simulink model "StarshotAC_DC_kd12"  (R2017a)
settings: Solver=FixedStepAuto  StartTime=0  StopTime=50000  FixedStep=0.01  MaxStep=4.0  MinStep=.001  RelTol=1e-6
values from neighbouring files (symbols this model uses):
  B0 = 3.12e-5    (= 3.12e-05)    [starshot_DC_KD_setup.m]    (also in starshot_DC_setup.m; starshotmath.m; temp.m)
  G = 6.67e-11    [starshot_DC_KD_setup.m]    (also in starshot_DC_setup.m; temp.m)
  M_Earth = 5.972e24    (= 5.972e+24)    [starshot_DC_KD_setup.m]    (also in starshot_DC_setup.m; temp.m)
  q0 = [qmatlab(2:4),qmatlab(1)]'    [starshot_DC_KD_setup.m]    (also in starshot_DC_setup.m; temp.m)
  R_Earth = 6.378e6    (= 6378000)    [starshot_DC_KD_setup.m]    (also in starshot_DC_setup.m; temp.m)
undefined symbols (not defined in the file or in its folder): starshot
libraries: dspmathops x1, sharedtransform x1, simulink x1
settings Model: Creator=armen  LastModifiedBy=Davide

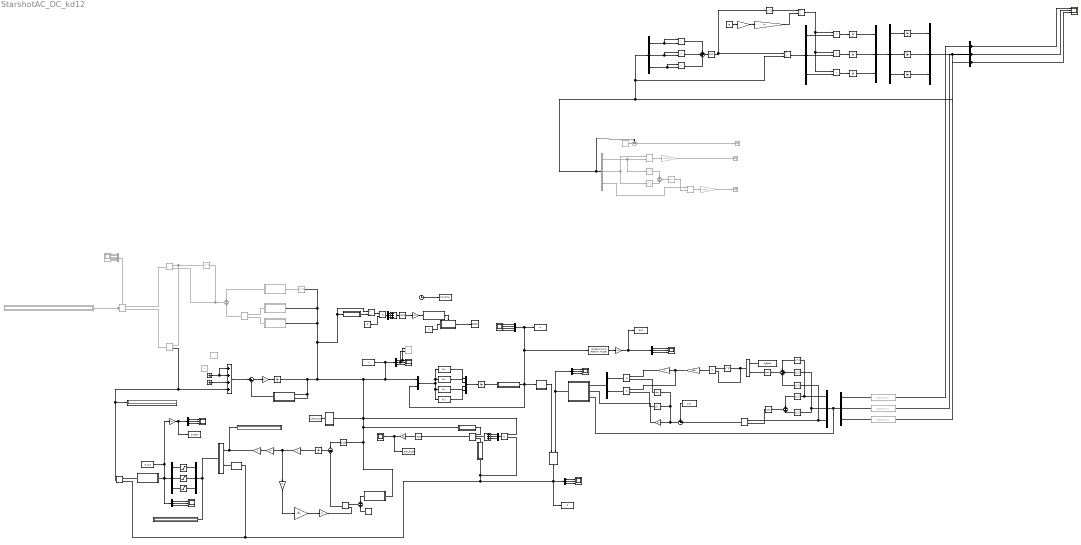
== system StarshotAC_DC_kd12 ==
  note: Dynamics
  note: Kynematics
  note: Earth's magnetic dipole
  note: Magnetic dipole/torque
  (w_b)x(L_b) : Subsystem
  Add : Sum  Inputs=3
  Add1 : Sum  Inputs=+++
  Angular velocity : Scope  NumInputPorts=3
  Clock : Clock
  Constant : Constant  Value=-G
  Constant1 : Constant  Value=R_Earth
  Constant2 : Constant  Commented=on  Value=[0;0;0]
  Constant3 : Constant  Value=starshot.IC.massproperties.PI(:,3)'
  Constant4 : Constant
  Constant5 : Constant  Commented=on  Value=starshot.IC.x
  Constant6 : Constant  Commented=on  Value=starshot.IC.y
  Constant7 : Constant  Commented=on  Value=starshot.IC.z
  Constant8 : Constant  Value=pi/2
  Cross : Subsystem
  Current : Scope  NumInputPorts=3
  Demux{,1..5,7..10,12,14,16,18} (14 alike) : Demux  Outputs=3
  Demux11 : Demux  Commented=on  Outputs=6
  Demux13 : Demux
  Demux6 : Demux  Commented=on  Outputs=3
  Derivative : Derivative
  Derivative1 : Derivative  Commented=on
  Dipole->ECI : Subsystem
  Display : Display  Commented=on
  Display1 : Display
  Display4 : Display
  Display6 : Display
  Divide : Product  Inputs=/*
  Divide1 : Product  Inputs=/*
  Divide2 : Product  Inputs=*/
  Divide3 : Product  Inputs=**
  Divide4 : Product  Inputs=**
  Divide5 : Product  Commented=on  Inputs=/*  Multiplication=Matrix(*)
  Divide6 : Product  Inputs=/*/
  Dot Product{,1..5} (6 alike) : DotProduct  InputSameDT=on  OutDataTypeStr=Inherit: Inherit via internal rule
  Earth's magnetic field (ECI) : Scope  NumInputPorts=3
  Earth's magnetic field (body) : Scope  NumInputPorts=3
  Euler angles : Scope  NumInputPorts=3
  Gain : Gain  Commented=on  Gain=180/pi
  Gain 1 : Gain  SaturateOnIntegerOverflow=on  OutDataTypeStr=Inherit: Same as input  ParamDataTypeStr=Inherit: Same as input
  Gain 2 : Gain  Gain=-1  SaturateOnIntegerOverflow=on  OutDataTypeStr=Inherit: Same as input  ParamDataTypeStr=Inherit: Same as input
  Gain 8 : Gain  Gain=starshot.cmd.c  SaturateOnIntegerOverflow=on  OutDataTypeStr=Inherit: Same as input  ParamDataTypeStr=Inherit: Same as input
  Gain 9 : Gain  Gain=-1  SaturateOnIntegerOverflow=on  OutDataTypeStr=Inherit: Same as input  ParamDataTypeStr=Inherit: Same as input
  Gain1 : Gain  Gain=M_Earth
  Gain18 : Gain  Gain=180/pi
  Gain2 : Gain  Gain=starshot.IC.massproperties.m
  Gain3 : Gain  Commented=on  Gain=180/pi
  Gain4 : Gain  Gain=-B0
  Gain5 : Gain  Gain=2
  Gain6 : Gain  Gain=-1
  Gain7 : Gain  Gain=1/0.0005
  Gain8 : Gain  Gain=180/pi
  Gain9 : Gain  Gain=180/pi
  Id inverse : Gain  Gain=starshot.cmd.invId  Multiplication=Matrix(K*u)  SaturateOnIntegerOverflow=on  OutDataTypeStr=Inherit: Same as input  ParamDataTypeStr=Inherit: Same as input
  Identity matrix : Constant  Value=[1 0 0;0 1 0;0 0 1]
  If : If  IfExpression=u1 < 0.2| u1>179.8  ShowElse=off
  If Action Subsystem : Subsystem  TreatAsAtomicUnit=on
  Integrator : Integrator  InitialCondition=starshot.IC.x
  Integrator1 : Integrator  InitialCondition=starshot.IC.y
  Integrator2 : Integrator  InitialCondition=starshot.IC.z
  Integrator3 : Integrator  InitialCondition=starshot.IC.xdot
  Integrator4 : Integrator  InitialCondition=starshot.IC.ydot
  Integrator5 : Integrator  InitialCondition=starshot.IC.zdot
  Integrator6 : Integrator  InitialCondition=starshot.IC.w
  Integrator7 : Integrator  InitialCondition=q0
  Integrator8 : Integrator  InitialCondition=starshot.cmd.wdb0
  Inv(I) : Gain  Gain=starshot.IC.massproperties.Iinv  Multiplication=Matrix(K*u)
  Kane damping : Gain  Gain=starshot.cmd.c  SaturateOnIntegerOverflow=on  OutDataTypeStr=Inherit: Same as input  ParamDataTypeStr=Inherit: Same as input
  L : Subsystem  Commented=on
  L1 : Subsystem  Commented=on
  Math Function{,3..8} (7 alike) : Math  Operator=square  SaturateOnIntegerOverflow=on
  Math Function1 : Math  Commented=on  Operator=square  SaturateOnIntegerOverflow=on
  Math Function2 : Math  Commented=on  Operator=square  SaturateOnIntegerOverflow=on
  Math Function9 : Math  Commented=on  Operator=transpose  SaturateOnIntegerOverflow=on
  Matrix Multiply : Product  Multiplication=Matrix(*)
  Mux{,1,6,9} (4 alike) : Mux  Inputs=3
  Mux10 : Mux
  Mux3 : Mux  Inputs=2
  Mux4 : Mux  Inputs=2
  Norm1 : Subsystem
  Norm4 : Subsystem
  Norm5 : Subsystem
  Normalization : dspmathops/Normalization  NormType=Squared 2-norm  Bias=1e-10  NormOver=Each column  Dimension=1  outputDataTypeStr=Inherit: Same as product output  outputLastDataTypeStr=Inherit: Same as product output  outputMin=[]  outputMax=[]  accumDataTypeStr=Inherit: Same as product output  accumLastDataTypeStr=Inherit: Same as product output  roundingMode=Floor  overflowMode=off
      settings: SourceProductName=DSP System Toolbox
  Normalized quat : Subsystem
  Product : Product
  Product1 : Product  Multiplication=Matrix(*)
  Product2 : Product  Multiplication=Matrix(*)
  Product3 : Product  Commented=on  Multiplication=Matrix(*)
  Product4 : Product  Commented=on  Multiplication=Matrix(*)
  Product5 : Product  Commented=on  Multiplication=Matrix(*)
  Product6 : Product
  Product7 : Product  Inputs=*/
  Product8 : Product
  Quaternion : Scope  NumInputPorts=4
  Quaternions to Rotation Angles : sharedtransform/Quaternions to Rotation Angles  rotationOrder=ZYX
  R_earth : Constant  Commented=on  Value=6.371e6
  Saturation : Saturate  UpperLimit=starshot.magnetorq.m_max_x  LowerLimit=-starshot.magnetorq.m_max_x
  Saturation1 : Saturate  UpperLimit=starshot.magnetorq.m_max_y  LowerLimit=-starshot.magnetorq.m_max_y
  Saturation2 : Saturate  UpperLimit=starshot.magnetorq.m_max_z  LowerLimit=-starshot.magnetorq.m_max_z
  Scope : Scope  NumInputPorts=3
  Scope1 : Scope  Commented=on  NumInputPorts=6
  Scope2 : Scope
  Skew matrix S(m) : Subsystem
  Skew matrix S(m)1 : Subsystem
  Skew matrix S(w) : Subsystem  Commented=on
  Sqrt : Sqrt  SaturateOnIntegerOverflow=on
  Sqrt1 : Sqrt  Commented=on  SaturateOnIntegerOverflow=on
  Sqrt2 : Sqrt  SaturateOnIntegerOverflow=on
  Sqrt3 : Sqrt  SaturateOnIntegerOverflow=on
  Stop Simulation : Stop
  Subsystem : Subsystem
  Sum : Sum  Inputs=+++
  Sum1 : Sum  Commented=on  Inputs=+-|
  Sum10 : Sum  Inputs=+|+  SaturateOnIntegerOverflow=on  InputSameDT=on  OutDataTypeStr=Inherit: Same as first input
  Sum12 : Sum  Inputs=|+-
  Sum2 : Sum  Commented=on
  Sum3 : Sum
  Sum4 : Sum  Inputs=+++
  Sum5 : Sum  Inputs=+-|
  Sum6 : Sum  Inputs=++++
  Sum7 : Sum  Commented=on  Inputs=+|+
  Sum8 : Sum  Inputs=--
  T_aero : Constant  Commented=on  Value=-starshot.aerodrag.Ta
  T_gravity : Ground
  T_solar : Ground
  Terminator : Terminator  Commented=on
  Terminator1 : Terminator  Commented=on
  Terminator2 : Terminator  Commented=on
  To Workspace : ToWorkspace  VariableName=real_angle  SaveFormat=Timeseries  SampleTime=-1
  To Workspace1 : ToWorkspace  VariableName=w  SaveFormat=Timeseries  SampleTime=-1
  To Workspace2 : ToWorkspace  VariableName=Eul1  SaveFormat=Timeseries  SampleTime=-1
  To Workspace3 : ToWorkspace  VariableName=w_error_out  SaveFormat=Timeseries  SampleTime=-1
  To Workspace4 : ToWorkspace  VariableName=b  SaveFormat=Timeseries  SampleTime=-1
  To Workspace5 : ToWorkspace  VariableName=m_out  SaveFormat=Timeseries  SampleTime=-1
  To Workspace6 : ToWorkspace  VariableName=q  SaveFormat=Timeseries  SampleTime=-1
  To Workspace7 : ToWorkspace  VariableName=current  SaveFormat=Timeseries  SampleTime=-1
  To Workspace8 : ToWorkspace  VariableName=sim_time  SaveFormat=Timeseries  SampleTime=-1
  Trigonometric Function : Trigonometry  Commented=on  Operator=atan2
  Trigonometric Function1 : Trigonometry  Commented=on  Operator=atan2
  Trigonometric Function2 : Trigonometry  Operator=cos
  Trigonometric Function3 : Trigonometry  Operator=atan2
  Trigonometric Function4 : Trigonometry
  Trigonometric Function5 : Trigonometry  Operator=acos
  Trigonometric Function6 : Trigonometry  Operator=acos
  XY Graph : simulink/Sinks/XY Graph  Commented=on  xmin=-2  xmax=2  ymin=-2  ymax=2  st=-1
  magnetic dipole : Scope  NumInputPorts=3
  qd(0) : Fcn  Expr=(u(7)*u(1)-u(6)*u(2)+u(5)*u(3))/2
  qd(1) : Fcn  Expr=(u(6)*u(1)+u(7)*u(2)-u(4)*u(3))/2
  qd(2) : Fcn  Expr=(-u(5)*u(1)+u(4)*u(2)+u(7)*u(3))/2
  qd(3) : Fcn  Expr=(-u(4)*u(1)-u(5)*u(2)-u(6)*u(3))/2
  quat to DCM : Subsystem  mask(Direction Cosine Matrix){}
      mask help: Determines the 3x3 Direction Cosine Matrix (DCM) from a 4x1 quaternion orientation vector. The outputted DCM transforms vectors from inertial axes to body axes. This version corrects the fucked-up MATLAB one.
      mask Help:
      | <p>This block determines the 3x3 Direction Cosine Matrix (DCM) from a 4x1 quaternion orientation vector. The outputted DCM transforms vectors from inertial axes to body axes.  This version corrects the fucked-up MATLAB one</p>
      | 
      | <p>The block input and output contain more than one signal as described below.</p>
      | 
      | <p><H4>Block Vector Input - Quaternion</H4>
      | <ul>
      | <li>q0</li>
      | <li>q1</li>
      | <li>q2</li>
      | <li>q3</li>
      | </ul>
      | </p>
      | 
      | <p><H4>Block Matrix Output - Direction Cosine Matrix  </H4>
      |     <ul>
      |    </ul>
      |    </p>
      mask Display: disp('q to Q')
  wires:
  Integrator/1 -> Mux/1
  Integrator2/1 -> Mux/3
  Integrator1/1 -> Mux/2
  Demux/3 -> Integrator2/1
  Demux/2 -> Integrator1/1
  Demux/1 -> Integrator/1
  Mux1/1 -> Demux/1
  Integrator5/1 -> Mux1/3
  Integrator4/1 -> Mux1/2
  Integrator3/1 -> Mux1/1
  Demux1/1 -> Dot Product/1, Dot Product/2
  Demux1/2 -> Dot Product1/1, Dot Product1/2
  Demux1/3 -> Dot Product2/1, Dot Product2/2
  Dot Product1/1 -> Sum/2
  Dot Product2/1 -> Sum/3
  Dot Product/1 -> Sum/1
  Sum/1 -> Sqrt/1
  Constant/1 -> Gain1/1
  Sqrt/1 -> Math Function/1, Divide1/1
  Gain1/1 -> Gain2/1
  Gain2/1 -> Divide/2
  Math Function/1 -> Divide/1
  Divide/1 -> Dot Product3/1, Dot Product4/1, Dot Product5/1
  Demux2/3 -> Dot Product3/2
  Demux2/2 -> Dot Product4/2
  Demux2/1 -> Dot Product5/2
  Dot Product5/1 -> Integrator3/1
  Dot Product4/1 -> Integrator4/1
  Dot Product3/1 -> Integrator5/1
  Divide1/1 -> Demux2/1
  Sum1/1 -> Terminator/1
  R_earth/1 -> Sum1/2
  Demux6/1 -> Math Function2/1, Trigonometric Function/2
  Demux6/2 -> Trigonometric Function/1, Math Function1/1
  Demux6/3 -> Trigonometric Function1/1
  Math Function2/1 -> Sum2/1
  Math Function1/1 -> Sum2/2
  Sum2/1 -> Sqrt1/1
  Sqrt1/1 -> Trigonometric Function1/2
  Trigonometric Function/1 -> Gain/1
  Trigonometric Function1/1 -> Gain3/1
  Gain/1 -> Terminator1/1
  Gain3/1 -> Terminator2/1
  Sqrt2/1 -> Trigonometric Function3/2
  Sum3/1 -> Sqrt2/1
  Math Function3/1 -> Sum3/2
  Math Function4/1 -> Sum3/1
  Demux7/3 -> Math Function7/1, Trigonometric Function3/1
  Demux7/2 -> Math Function3/1, Math Function6/1
  Demux7/1 -> Math Function5/1, Math Function4/1
  Mux/1 -> Sum1/1, Demux6/1, Divide1/2, Demux1/1, Demux3/1
  Math Function6/1 -> Sum4/2
  Math Function5/1 -> Sum4/1
  Math Function7/1 -> Sum4/3
  Sum4/1 -> Sqrt3/1
  Sqrt3/1 -> Divide2/2
  Constant1/1 -> Divide2/1
  Divide2/1 -> Product/2, Math Function8/1
  Math Function8/1 -> Product/1
  Product/1 -> Gain4/1
  Gain4/1 -> Divide4/1, Gain5/1
  Gain5/1 -> Divide3/1
  Trigonometric Function2/1 -> Divide3/2
  Trigonometric Function4/1 -> Divide4/2
  Divide3/1 -> Mux4/1
  Divide4/1 -> Mux4/2
  Mux4/1 -> Dipole->ECI/1(B_r,B_theta)
  Gain6/1 -> Dipole->ECI/2(-theta)
  Demux9/3 -> Earth's magnetic field (ECI)/3
  Demux9/1 -> Earth's magnetic field (ECI)/1
  Demux9/2 -> Earth's magnetic field (ECI)/2
  Mux6/1 -> Dipole->ECI/3(r), Demux7/1
  Demux3/3 -> Scope/3, Mux6/3
  Demux3/2 -> Scope/2, Mux6/2
  Demux3/1 -> Scope/1, Mux6/1
  Trigonometric Function3/1 -> Sum5/2
  Constant8/1 -> Sum5/1
  Sum5/1 -> Trigonometric Function2/1, Trigonometric Function4/1, Gain6/1
  Demux13/1 -> Quaternion/1
  Demux13/4 -> Quaternion/4
  Demux13/3 -> Quaternion/3
  Demux13/2 -> Quaternion/2
  Demux16/2 -> XY Graph/2, Angular velocity/2
  Demux16/1 -> XY Graph/1, Angular velocity/1
  Demux16/3 -> Angular velocity/3
  Dipole->ECI/1(B) -> Demux9/1, Matrix Multiply/2
  Demux8/1 -> Saturation/1
  Saturation2/1 -> Mux9/3
  Saturation/1 -> Mux9/1
  Demux8/2 -> Saturation1/1
  Saturation1/1 -> Mux9/2
  Demux10/3 -> magnetic dipole/3
  Demux10/2 -> magnetic dipole/2
  Demux10/1 -> magnetic dipole/1
  quat to DCM/1(DCM) -> Matrix Multiply/1
  Demux18/3 -> Euler angles/3
  Demux18/1 -> Euler angles/1
  Gain18/1 -> To Workspace2/1, Demux18/1  "Euler Angles plot"
  Quaternions to Rotation Angles/1 -> Gain18/1
  Demux18/2 -> Euler angles/2
  Inv(I)/1 -> Integrator6/1
  (w_b)x(L_b)/1((w_b)x(L_b)) -> Sum12/2
  Sum12/1 -> Inv(I)/1  "wdot"
  qd(2)/1 -> Mux10/3
  qd(1)/1 -> Mux10/2
  Normalized quat/1(q^) -> Mux3/2, quat to DCM/1(e0 e1 e2 e3), Quaternions to Rotation Angles/1, To Workspace6/1, Demux13/1  "q^"
  qd(3)/1 -> Mux10/4
  Integrator7/1 -> Normalized quat/1(q)
  Mux10/1 -> Integrator7/1
  qd(0)/1 -> Mux10/1
  Mux3/1 -> qd(3)/1, qd(2)/1, qd(1)/1, qd(0)/1
  Demux4/1 -> Earth's magnetic field (body)/1
  Demux4/2 -> Earth's magnetic field (body)/2
  Demux4/3 -> Earth's magnetic field (body)/3
  T_gravity/1 -> Sum6/1, Sum6/2
  Sum6/1 -> Sum12/1
  Mux9/1 -> Skew matrix S(m)/1(m), To Workspace5/1, Gain7/1, Demux10/1
  Gain7/1 -> To Workspace7/1, Demux5/1
  Demux5/1 -> Current/1
  Demux5/2 -> Current/2
  Demux5/3 -> Current/3
  Skew matrix S(m)/1(S(m)) -> Product2/1
  Demux8/3 -> Saturation2/1
  Cross/1(AxB) -> Display6/1, Demux8/1
  Product2/1 -> Product4/2, Sum6/4, Display4/1
  Gain 2/1 -> Kane damping/1, Gain 9/1
  Normalization/1 -> Cross/2(B)
  Kane damping/1 -> Gain 1/1
  Derivative/1 -> Sum8/1
  Sum8/1 -> Integrator8/1
  Gain 8/1 -> Product1/2
  Id inverse/1 -> Gain 8/1
  Skew matrix S(m)1/1(S(w)) -> Sum10/1
  Identity matrix/1 -> Sum10/2
  Gain 9/1 -> Id inverse/1
  Sum10/1 -> Product1/1
  Product1/1 -> Sum8/2
  Gain 1/1 -> Display1/1, Cross/1(A)
  Integrator8/1 -> Gain 2/1  "w_(d/b)"
  Divide5/1 -> Display/1, Demux11/1
  Sum7/1 -> Product3/2, Math Function9/1
  Math Function9/1 -> Product4/1, Product3/1
  Product3/1 -> Divide5/1
  Product4/1 -> Divide5/2
  Demux11/1 -> Scope1/1
  Demux11/2 -> Scope1/2
  Demux11/3 -> Scope1/3
  Demux11/4 -> Scope1/4
  Demux11/5 -> Scope1/5
  Demux11/6 -> Scope1/6
  L1/1(L(a)) -> Product5/2
  Skew matrix S(w)/1(S(w)) -> Product5/1
  L/1(L(a)) -> Sum7/1
  Product5/1 -> Sum7/2
  Derivative1/1 -> L/1(a)
  Demux12/3 -> Add/3
  Divide6/1 -> Trigonometric Function5/1
  Norm5/1(norm(v)) -> Divide6/3
  Add/1 -> Divide6/2
  Matrix Multiply/1 -> To Workspace4/1, Demux4/1, Product6/2, Norm5/1(v), Normalization/1, Product2/2
  Demux12/1 -> Add/1
  Demux12/2 -> Add/2
  Integrator6/1 -> Product7/1, Norm1/1(v), Derivative1/1, Skew matrix S(w)/1(w), L1/1(a), Subsystem/1(In1), Norm4/1(v), Skew matrix S(m)1/1(w), Derivative/1, Product6/1, Mux3/1, Demux16/1, To Workspace1/1, (w_b)x(L_b)/2(L_b), (w_b)x(L_b)/1(w_b)  "w"
  Product6/1 -> Demux12/1
  Trigonometric Function5/1 -> Gain8/1
  Norm4/1(norm(v)) -> Divide6/1
  Gain8/1 -> To Workspace/1, Scope2/1
  Subsystem/1(Out1) -> To Workspace3/1
  T_solar/1 -> Sum6/3
  Constant3/1 -> Product8/2
  Norm1/1(norm(v)) -> Product7/2
  Trigonometric Function6/1 -> Gain9/1
  Gain9/1 -> If/1
  Product7/1 -> Product8/1
  If/1 -> If Action Subsystem/Action
  Constant4/1 -> If Action Subsystem/1(In1)
  If Action Subsystem/1(Out1) -> Stop Simulation/1
  Add1/1 -> Trigonometric Function6/1
  Product8/1 -> Demux14/1
  Demux14/1 -> Add1/1
  Demux14/2 -> Add1/2
  Demux14/3 -> Add1/3
  Clock/1 -> To Workspace8/1

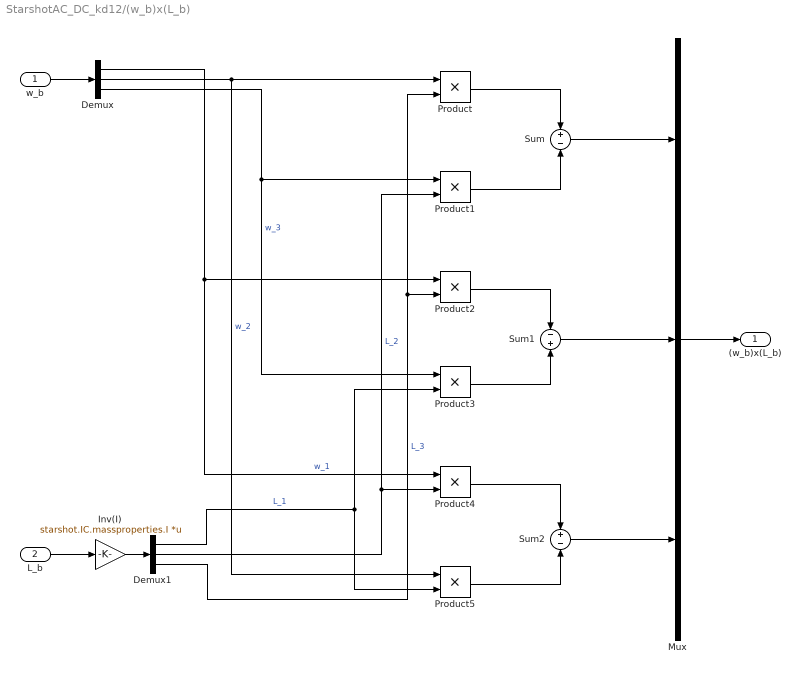
== system StarshotAC_DC_kd12/(w_b)x(L_b) ==
  w_b : Inport
  L_b : Inport  Port=2
  Demux : Demux  Outputs=3
  Demux1 : Demux  Outputs=3
  Inv(I) : Gain  Gain=starshot.IC.massproperties.I  Multiplication=Matrix(K*u)
  Mux : Mux  Inputs=3
  Product{,1..5} (6 alike) : Product
  Sum : Sum  Inputs=+|-
  Sum1 : Sum  Inputs=-|+
  Sum2 : Sum  Inputs=+|-
  (w_b)x(L_b) : Outport
  wires:
  w_b/1 -> Demux/1
  L_b/1 -> Inv(I)/1
  Demux/3 -> Product1/1, Product3/1  "w_3"
  Demux/2 -> Product5/1, Product/1  "w_2"
  Demux/1 -> Product2/1, Product4/1  "w_1"
  Mux/1 -> (w_b)x(L_b)/1
  Demux1/3 -> Product2/2, Product/2  "L_3"
  Demux1/2 -> Product1/2, Product4/2  "L_2"
  Product1/1 -> Sum/2
  Product/1 -> Sum/1
  Demux1/1 -> Product5/2, Product3/2  "L_1"
  Sum/1 -> Mux/1
  Sum2/1 -> Mux/3
  Sum1/1 -> Mux/2
  Product5/1 -> Sum2/2
  Product4/1 -> Sum2/1
  Product3/1 -> Sum1/2
  Product2/1 -> Sum1/1
  Inv(I)/1 -> Demux1/1

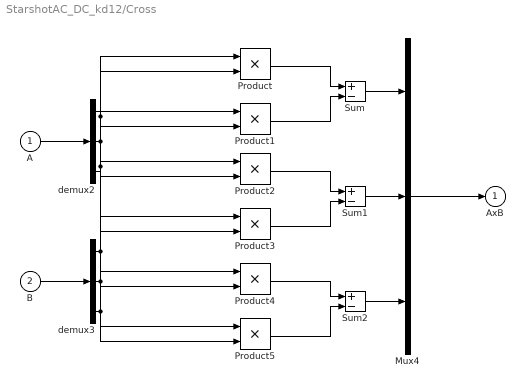
== system StarshotAC_DC_kd12/Cross ==
  A : Inport
  B : Inport  Port=2
  Mux4 : Mux  Inputs=3
  Product{,1..5} (6 alike) : Product  SaturateOnIntegerOverflow=on  InputSameDT=on  OutDataTypeStr=Inherit: Same as first input
  Sum : Sum  Inputs=+-  SaturateOnIntegerOverflow=on  InputSameDT=on  OutDataTypeStr=Inherit: Same as first input
  Sum1 : Sum  Inputs=+-  SaturateOnIntegerOverflow=on  InputSameDT=on  OutDataTypeStr=Inherit: Same as first input
  Sum2 : Sum  Inputs=+-  SaturateOnIntegerOverflow=on  InputSameDT=on  OutDataTypeStr=Inherit: Same as first input
  demux2 : Demux  Outputs=3
  demux3 : Demux  Outputs=3
  AxB : Outport  InitialOutput=0
  wires:
  A/1 -> demux2/1
  B/1 -> demux3/1
  demux2/3 -> Product1/1, Product2/1
  demux3/3 -> Product/2, Product3/2
  demux2/1 -> Product3/1, Product4/1
  demux3/2 -> Product1/2, Product4/2
  demux2/2 -> Product/1, Product5/1
  demux3/1 -> Product2/2, Product5/2
  Product/1 -> Sum/1
  Product1/1 -> Sum/2
  Product2/1 -> Sum1/1
  Product3/1 -> Sum1/2
  Product4/1 -> Sum2/1
  Product5/1 -> Sum2/2
  Sum/1 -> Mux4/1
  Sum1/1 -> Mux4/2
  Sum2/1 -> Mux4/3
  Mux4/1 -> AxB/1

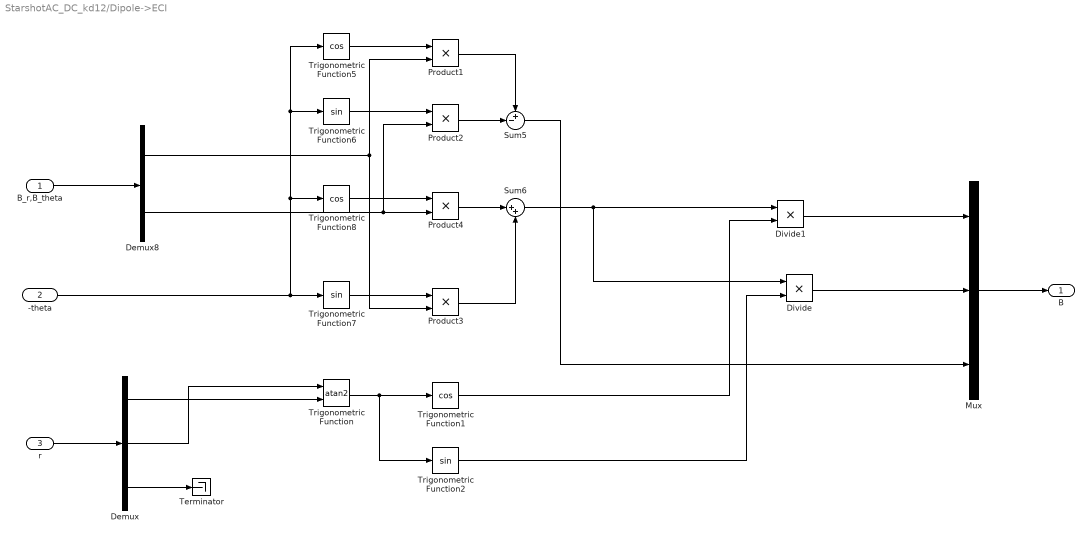
== system StarshotAC_DC_kd12/Dipole->ECI ==
  B_r,B_theta : Inport
  -theta : Inport  Port=2
  r : Inport  Port=3
  Demux : Demux  Outputs=3
  Demux8 : Demux  Outputs=2
  Divide : Product  Inputs=**
  Divide1 : Product  Inputs=**
  Mux : Mux  Inputs=3
  Product{1..4} (4 alike) : Product
  Sum5 : Sum  Inputs=+-|
  Sum6 : Sum  Inputs=|++
  Terminator : Terminator
  Trigonometric Function : Trigonometry  Operator=atan2
  Trigonometric Function1 : Trigonometry  Operator=cos
  Trigonometric Function2 : Trigonometry
  Trigonometric Function5 : Trigonometry  Operator=cos
  Trigonometric Function6 : Trigonometry
  Trigonometric Function7 : Trigonometry
  Trigonometric Function8 : Trigonometry  Operator=cos
  B : Outport
  wires:
  -theta/1 -> Trigonometric Function5/1, Trigonometric Function6/1, Trigonometric Function8/1, Trigonometric Function7/1
  Product4/1 -> Sum6/1
  Product3/1 -> Sum6/2
  Demux8/1 -> Product3/2, Product1/2
  Demux8/2 -> Product2/2, Product4/2
  Trigonometric Function5/1 -> Product1/1
  Product2/1 -> Sum5/2
  Trigonometric Function7/1 -> Product3/1
  B_r,B_theta/1 -> Demux8/1
  Sum5/1 -> Mux/3
  Trigonometric Function8/1 -> Product4/1
  Trigonometric Function6/1 -> Product2/1
  Sum6/1 -> Divide1/1, Divide/1
  Product1/1 -> Sum5/1
  r/1 -> Demux/1
  Demux/3 -> Terminator/1
  Demux/2 -> Trigonometric Function/1
  Demux/1 -> Trigonometric Function/2
  Trigonometric Function/1 -> Trigonometric Function1/1, Trigonometric Function2/1
  Trigonometric Function1/1 -> Divide1/2
  Trigonometric Function2/1 -> Divide/2
  Mux/1 -> B/1
  Divide1/1 -> Mux/1
  Divide/1 -> Mux/2

== system StarshotAC_DC_kd12/If Action Subsystem ==
  In1 : Inport
  Action Port : ActionPort  ActionType=then
  Out1 : Outport
  wires:
  In1/1 -> Out1/1

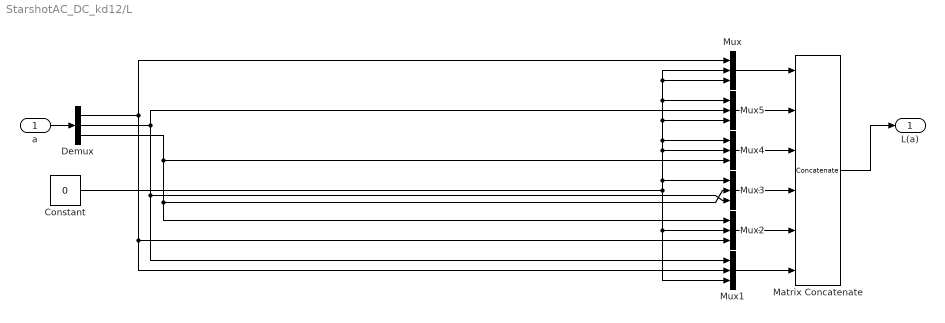
== system StarshotAC_DC_kd12/L ==
  a : Inport
  Constant : Constant  Value=0
  Demux : Demux  Outputs=3
  Matrix Concatenate : Concatenate  NumInputs=6  Mode=Multidimensional array  ConcatenateDimension=2
  Mux{,1..5} (6 alike) : Mux  Inputs=3
  L(a) : Outport
  wires:
  a/1 -> Demux/1
  Matrix Concatenate/1 -> L(a)/1
  Mux/1 -> Matrix Concatenate/1
  Mux5/1 -> Matrix Concatenate/2
  Mux4/1 -> Matrix Concatenate/3
  Mux3/1 -> Matrix Concatenate/4
  Mux2/1 -> Matrix Concatenate/5
  Mux1/1 -> Matrix Concatenate/6
  Demux/1 -> Mux1/2, Mux2/3, Mux/1
  Constant/1 -> Mux1/3, Mux2/2, Mux3/1, Mux4/2, Mux4/1, Mux5/3, Mux5/1, Mux/2, Mux/3
  Demux/2 -> Mux1/1, Mux3/3, Mux5/2
  Demux/3 -> Mux2/1, Mux3/2, Mux4/3

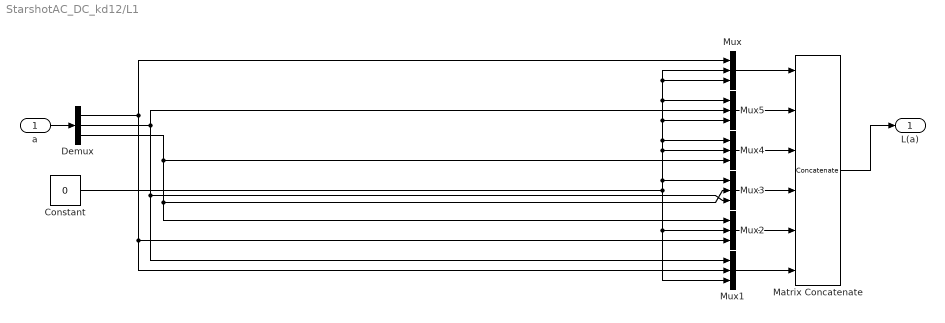
== system StarshotAC_DC_kd12/L1 ==
  a : Inport
  Constant : Constant  Value=0
  Demux : Demux  Outputs=3
  Matrix Concatenate : Concatenate  NumInputs=6  Mode=Multidimensional array  ConcatenateDimension=2
  Mux{,1..5} (6 alike) : Mux  Inputs=3
  L(a) : Outport
  wires:
  a/1 -> Demux/1
  Matrix Concatenate/1 -> L(a)/1
  Mux/1 -> Matrix Concatenate/1
  Mux5/1 -> Matrix Concatenate/2
  Mux4/1 -> Matrix Concatenate/3
  Mux3/1 -> Matrix Concatenate/4
  Mux2/1 -> Matrix Concatenate/5
  Mux1/1 -> Matrix Concatenate/6
  Demux/1 -> Mux1/2, Mux2/3, Mux/1
  Constant/1 -> Mux1/3, Mux2/2, Mux3/1, Mux4/2, Mux4/1, Mux5/3, Mux5/1, Mux/2, Mux/3
  Demux/2 -> Mux1/1, Mux3/3, Mux5/2
  Demux/3 -> Mux2/1, Mux3/2, Mux4/3

== system StarshotAC_DC_kd12/Norm1 ==
  v : Inport
  Dot Product6 : DotProduct  InputSameDT=on  OutDataTypeStr=Inherit: Inherit via internal rule
  Sqrt4 : Sqrt  SaturateOnIntegerOverflow=on
  norm(v) : Outport
  wires:
  v/1 -> Dot Product6/1, Dot Product6/2
  Dot Product6/1 -> Sqrt4/1
  Sqrt4/1 -> norm(v)/1

== system StarshotAC_DC_kd12/Norm4 ==
  v : Inport
  Dot Product6 : DotProduct  InputSameDT=on  OutDataTypeStr=Inherit: Inherit via internal rule
  Sqrt4 : Sqrt  SaturateOnIntegerOverflow=on
  norm(v) : Outport
  wires:
  v/1 -> Dot Product6/1, Dot Product6/2
  Dot Product6/1 -> Sqrt4/1
  Sqrt4/1 -> norm(v)/1

== system StarshotAC_DC_kd12/Norm5 ==
  v : Inport
  Dot Product6 : DotProduct  InputSameDT=on  OutDataTypeStr=Inherit: Inherit via internal rule
  Sqrt4 : Sqrt  SaturateOnIntegerOverflow=on
  norm(v) : Outport
  wires:
  v/1 -> Dot Product6/1, Dot Product6/2
  Dot Product6/1 -> Sqrt4/1
  Sqrt4/1 -> norm(v)/1

== system StarshotAC_DC_kd12/Normalized quat ==
  q : Inport
  Modulo1 : Subsystem
  Product2 : Product  Inputs=*/  SaturateOnIntegerOverflow=on  OutDataTypeStr=Inherit: Same as first input
  q^ : Outport
  wires:
  q/1 -> Modulo1/1(q), Product2/1
  Modulo1/1(Module q) -> Product2/2
  Product2/1 -> q^/1

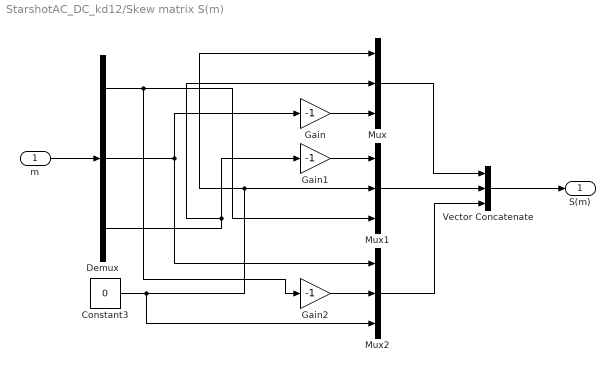
== system StarshotAC_DC_kd12/Skew matrix S(m) ==
  m : Inport
  Constant3 : Constant  Value=0
  Demux : Demux  Outputs=3
  Gain : Gain  Gain=-1
  Gain1 : Gain  Gain=-1
  Gain2 : Gain  Gain=-1
  Mux : Mux  Inputs=3
  Mux1 : Mux  Inputs=3
  Mux2 : Mux  Inputs=3
  Vector Concatenate : Concatenate  NumInputs=3  Mode=Multidimensional array  ConcatenateDimension=2
  S(m) : Outport
  wires:
  Gain/1 -> Mux/3
  Demux/2 -> Mux2/1, Gain/1
  Demux/3 -> Gain1/1, Mux/2
  Gain2/1 -> Mux2/2
  Demux/1 -> Mux1/3, Gain2/1
  Mux1/1 -> Vector Concatenate/2
  m/1 -> Demux/1
  Constant3/1 -> Mux2/3, Mux/1, Mux1/2
  Vector Concatenate/1 -> S(m)/1
  Mux/1 -> Vector Concatenate/1
  Mux2/1 -> Vector Concatenate/3
  Gain1/1 -> Mux1/1

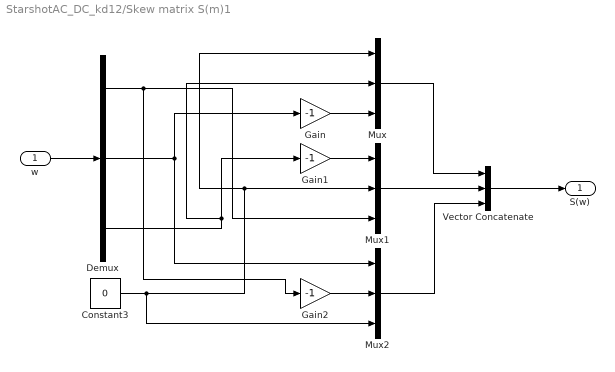
== system StarshotAC_DC_kd12/Skew matrix S(m)1 ==
  w : Inport
  Constant3 : Constant  Value=0
  Demux : Demux  Outputs=3
  Gain : Gain  Gain=-1
  Gain1 : Gain  Gain=-1
  Gain2 : Gain  Gain=-1
  Mux : Mux  Inputs=3
  Mux1 : Mux  Inputs=3
  Mux2 : Mux  Inputs=3
  Vector Concatenate : Concatenate  NumInputs=3  Mode=Multidimensional array  ConcatenateDimension=2
  S(w) : Outport
  wires:
  Gain/1 -> Mux/3
  Demux/2 -> Mux2/1, Gain/1
  Demux/3 -> Gain1/1, Mux/2
  Gain2/1 -> Mux2/2
  Demux/1 -> Mux1/3, Gain2/1
  Mux1/1 -> Vector Concatenate/2
  w/1 -> Demux/1
  Constant3/1 -> Mux2/3, Mux/1, Mux1/2
  Vector Concatenate/1 -> S(w)/1
  Mux/1 -> Vector Concatenate/1
  Mux2/1 -> Vector Concatenate/3
  Gain1/1 -> Mux1/1

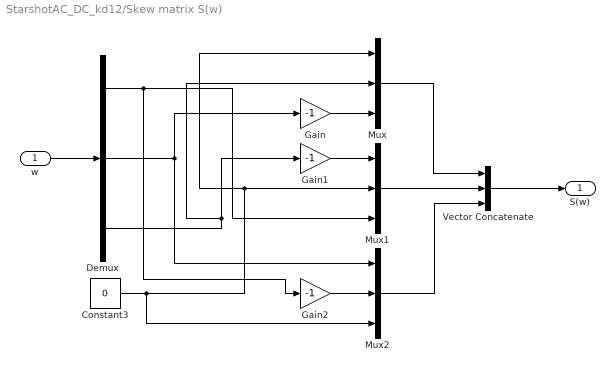
== system StarshotAC_DC_kd12/Skew matrix S(w) ==
  w : Inport
  Constant3 : Constant  Value=0
  Demux : Demux  Outputs=3
  Gain : Gain  Gain=-1
  Gain1 : Gain  Gain=-1
  Gain2 : Gain  Gain=-1
  Mux : Mux  Inputs=3
  Mux1 : Mux  Inputs=3
  Mux2 : Mux  Inputs=3
  Vector Concatenate : Concatenate  NumInputs=3  Mode=Multidimensional array  ConcatenateDimension=2
  S(w) : Outport
  wires:
  Gain/1 -> Mux/3
  Demux/2 -> Mux2/1, Gain/1
  Demux/3 -> Gain1/1, Mux/2
  Gain2/1 -> Mux2/2
  Demux/1 -> Mux1/3, Gain2/1
  Mux1/1 -> Vector Concatenate/2
  w/1 -> Demux/1
  Constant3/1 -> Mux2/3, Mux/1, Mux1/2
  Vector Concatenate/1 -> S(w)/1
  Mux/1 -> Vector Concatenate/1
  Mux2/1 -> Vector Concatenate/3
  Gain1/1 -> Mux1/1

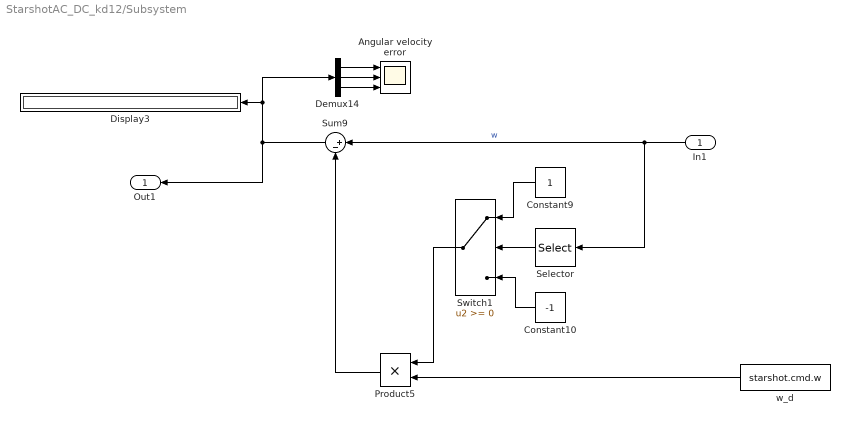
== system StarshotAC_DC_kd12/Subsystem ==
  In1 : Inport
  Angular velocity error : Scope  NumInputPorts=3
  Constant10 : Constant  Value=-1
  Constant9 : Constant
  Demux14 : Demux  Outputs=3
  Display3 : Display
  Product5 : Product  Inputs=**
  Selector : Selector  InputPortWidth=3  IndexOptions=Index vector (dialog)  Indices=[3]  OutputSizes=1
  Sum9 : Sum  Inputs=|+-
  Switch1 : Switch  ZeroCross=off
  w_d : Constant  Value=starshot.cmd.w
  Out1 : Outport
  wires:
  Product5/1 -> Sum9/2
  w_d/1 -> Product5/2
  Demux14/1 -> Angular velocity error/1
  Sum9/1 -> Out1/1, Demux14/1, Display3/1
  Demux14/3 -> Angular velocity error/3
  Demux14/2 -> Angular velocity error/2
  Selector/1 -> Switch1/2
  Constant10/1 -> Switch1/3
  Constant9/1 -> Switch1/1
  In1/1 -> Selector/1, Sum9/1  "w"
  Switch1/1 -> Product5/1

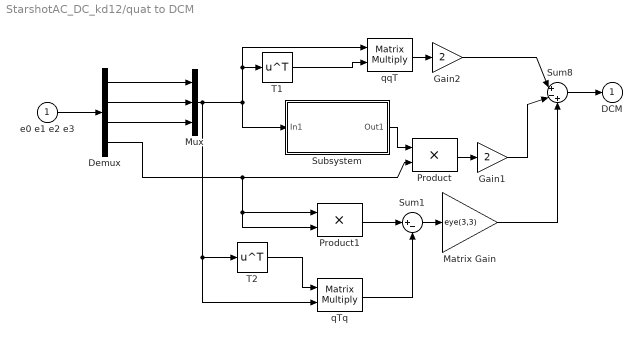
== system StarshotAC_DC_kd12/quat to DCM ==
  e0 e1 e2 e3 : Inport
  Demux : Demux
  Gain1 : Gain  Gain=2  SaturateOnIntegerOverflow=on  OutDataTypeStr=Inherit: Same as input  ParamDataTypeStr=Inherit: Same as input
  Gain2 : Gain  Gain=2  SaturateOnIntegerOverflow=on  OutDataTypeStr=Inherit: Same as input  ParamDataTypeStr=Inherit: Same as input
  Matrix Gain : Gain  Gain=eye(3,3)  SaturateOnIntegerOverflow=on  OutDataTypeStr=Inherit: Same as input  ParamDataTypeStr=Inherit: Same as input
  Mux : Mux  Inputs=3
  Product : Product  SaturateOnIntegerOverflow=on  InputSameDT=on  OutDataTypeStr=Inherit: Same as first input
  Product1 : Product  SaturateOnIntegerOverflow=on  InputSameDT=on  OutDataTypeStr=Inherit: Same as first input
  Subsystem : Subsystem
      mask Display: disp('3x3 cross matrix')
  Sum1 : Sum  Inputs=|+-  SaturateOnIntegerOverflow=on  InputSameDT=on  OutDataTypeStr=Inherit: Same as first input
  Sum8 : Sum  Inputs=|+-+  SaturateOnIntegerOverflow=on  InputSameDT=on  OutDataTypeStr=Inherit: Same as first input
  T1 : Math  Operator=transpose  SaturateOnIntegerOverflow=on
  T2 : Math  Operator=transpose  SaturateOnIntegerOverflow=on
  qTq : Product  Multiplication=Matrix(*)  SaturateOnIntegerOverflow=on  InputSameDT=on  OutDataTypeStr=Inherit: Same as first input
  qqT : Product  Multiplication=Matrix(*)  SaturateOnIntegerOverflow=on  InputSameDT=on  OutDataTypeStr=Inherit: Same as first input
  DCM : Outport  InitialOutput=0
  wires:
  Subsystem/1(Out1) -> Product/1
  Matrix Gain/1 -> Sum8/3
  Sum1/1 -> Matrix Gain/1
  qTq/1 -> Sum1/2
  T2/1 -> qTq/1
  Product1/1 -> Sum1/1
  Gain1/1 -> Sum8/2
  Gain2/1 -> Sum8/1
  qqT/1 -> Gain2/1
  T1/1 -> qqT/2
  Product/1 -> Gain1/1
  Mux/1 -> qTq/2, T2/1, qqT/1, T1/1, Subsystem/1(In1)
  Demux/4 -> Product1/2, Product1/1, Product/2
  Demux/3 -> Mux/3
  Demux/2 -> Mux/2
  Demux/1 -> Mux/1
  e0 e1 e2 e3/1 -> Demux/1
  Sum8/1 -> DCM/1

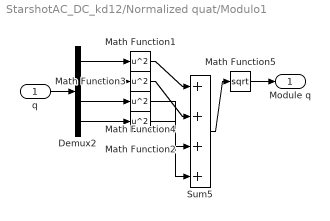
== system StarshotAC_DC_kd12/Normalized quat/Modulo1 ==
  q : Inport
  Demux2 : Demux
  Math Function{1..4} (4 alike) : Math  Operator=square  SaturateOnIntegerOverflow=on
  Math Function5 : Math  Operator=sqrt  SaturateOnIntegerOverflow=on
  Sum5 : Sum  Inputs=|++++  SaturateOnIntegerOverflow=on
  Module q : Outport
  wires:
  q/1 -> Demux2/1
  Math Function5/1 -> Module q/1
  Sum5/1 -> Math Function5/1
  Math Function4/1 -> Sum5/3
  Math Function3/1 -> Sum5/2
  Math Function1/1 -> Sum5/1
  Demux2/3 -> Math Function4/1
  Demux2/2 -> Math Function3/1
  Demux2/1 -> Math Function1/1
  Demux2/4 -> Math Function2/1
  Math Function2/1 -> Sum5/4

== system StarshotAC_DC_kd12/quat to DCM/Subsystem ==
  In1 : Inport
  3x3 : Reshape  OutputDimensionality=Customize  OutputDimensions=[3,3]
  Demux : Demux  Outputs=3
  Gain : Gain  Gain=-1  SaturateOnIntegerOverflow=on  OutDataTypeStr=Inherit: Same as input  ParamDataTypeStr=Inherit: Same as input
  Gain1 : Gain  Gain=-1  SaturateOnIntegerOverflow=on  OutDataTypeStr=Inherit: Same as input  ParamDataTypeStr=Inherit: Same as input
  Gain2 : Gain  Gain=-1  SaturateOnIntegerOverflow=on  OutDataTypeStr=Inherit: Same as input  ParamDataTypeStr=Inherit: Same as input
  Mux : Mux  Inputs=9
  "diag 0 " : Constant  Value=0
  Out1 : Outport
  wires:
  Gain2/1 -> Mux/8
  Demux/1 -> Gain2/1, Mux/6
  Gain1/1 -> Mux/4
  Demux/2 -> Mux/7, Gain/1
  Gain/1 -> Mux/3
  Demux/3 -> Gain1/1, Mux/2
  Mux/1 -> 3x3/1
  "diag 0 "/1 -> Mux/9, Mux/5, Mux/1
  3x3/1 -> Out1/1
  In1/1 -> Demux/1
